simulink model "DC_PlugIn_FastCharging"  (R2023b)
settings: Solver=FixedStepAuto  StartTime=0.0  StopTime=10.0  FixedStep=0.001  RelTol=1e-3
settings Model: Creator=OWNER  LastModifiedBy=OWNER

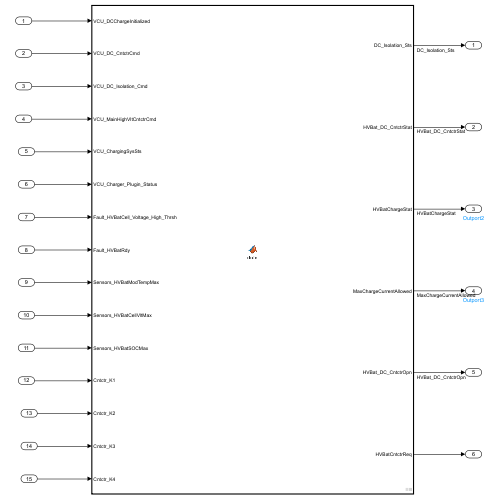
[thumbnail: Simulink's stored preview of the top-level diagram]
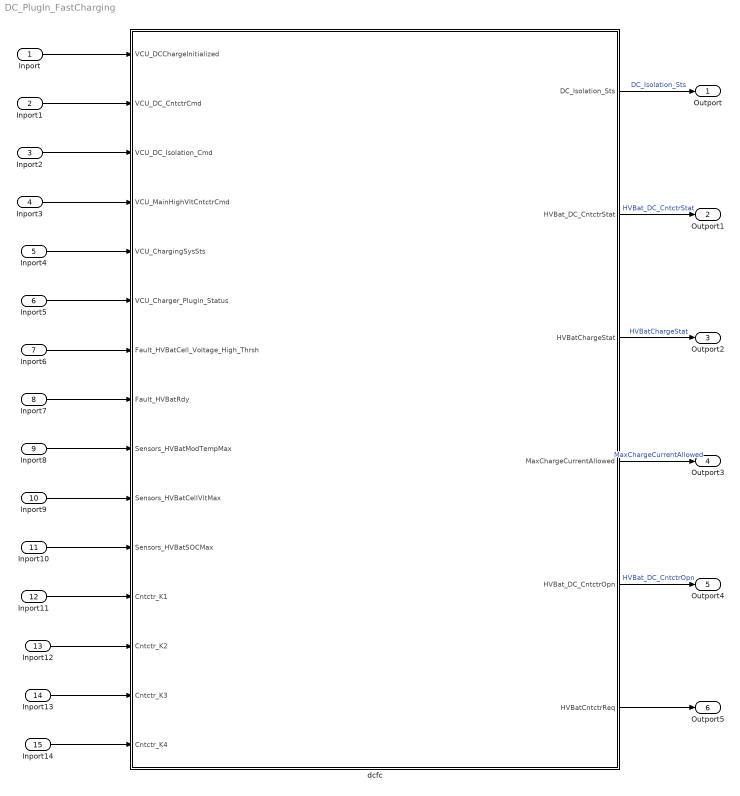
== system DC_PlugIn_FastCharging ==
  Inport : Inport
  Inport1 : Inport  Port=2
  Inport2 : Inport  Port=3
  Inport3 : Inport  Port=4
  Inport4 : Inport  Port=5
  Inport5 : Inport  Port=6
  Inport6 : Inport  Port=7
  Inport7 : Inport  Port=8
  Inport8 : Inport  Port=9
  Inport9 : Inport  Port=10
  Inport10 : Inport  Port=11
  Inport11 : Inport  Port=12
  Inport12 : Inport  Port=13
  Inport13 : Inport  Port=14
  Inport14 : Inport  Port=15
  dcfc : MATLAB Function  TreatAsAtomicUnit=on
  Outport : Outport
  Outport1 : Outport  Port=2
  Outport2 : Outport  Port=3
  Outport3 : Outport  Port=4
  Outport4 : Outport  Port=5
  Outport5 : Outport  Port=6
  wires:
  dcfc/1(DC_Isolation_Sts) -> Outport/1  "DC_Isolation_Sts"
  dcfc/2(HVBat_DC_CntctrStat) -> Outport1/1  "HVBat_DC_CntctrStat"
  dcfc/3(HVBatChargeStat) -> Outport2/1  "HVBatChargeStat"
  dcfc/4(MaxChargeCurrentAllowed) -> Outport3/1  "MaxChargeCurrentAllowed"
  dcfc/5(HVBat_DC_CntctrOpn) -> Outport4/1  "HVBat_DC_CntctrOpn"
  dcfc/6(HVBatCntctrReq) -> Outport5/1
  Inport/1 -> dcfc/1(VCU_DCChargeInitialized)
  Inport1/1 -> dcfc/2(VCU_DC_CntctrCmd)
  Inport2/1 -> dcfc/3(VCU_DC_Isolation_Cmd)
  Inport3/1 -> dcfc/4(VCU_MainHighVltCntctrCmd)
  Inport4/1 -> dcfc/5(VCU_ChargingSysSts)
  Inport7/1 -> dcfc/8(Fault_HVBatRdy)
  Inport6/1 -> dcfc/7(Fault_HVBatCell_Voltage_High_Thrsh)
  Inport5/1 -> dcfc/6(VCU_Charger_Plugin_Status)
  Inport8/1 -> dcfc/9(Sensors_HVBatModTempMax)
  Inport11/1 -> dcfc/12(Cntctr_K1)
  Inport10/1 -> dcfc/11(Sensors_HVBatSOCMax)
  Inport9/1 -> dcfc/10(Sensors_HVBatCellVltMax)
  Inport13/1 -> dcfc/14(Cntctr_K3)
  Inport12/1 -> dcfc/13(Cntctr_K2)
  Inport14/1 -> dcfc/15(Cntctr_K4)

== matlab function DC_PlugIn_FastCharging/dcfc ==
  settings: updateMethod=DISCRETE
  data: DC_Isolation_Sts output; HVBat_DC_CntctrStat output; HVBatChargeStat output; VCU_DCChargeInitialized input; MaxChargeCurrentAllowed output; VCU_DC_CntctrCmd input; VCU_DC_Isolation_Cmd input; VCU_MainHighVltCntctrCmd input; VCU_ChargingSysSts input; VCU_Charger_Plugin_Status input; Fault_HVBatCell_Voltage_High_Thrsh input; Fault_HVBatRdy input; Sensors_HVBatModTempMax input; Sensors_HVBatCellVltMax input; Sensors_HVBatSOCMax input; Cntctr_K1 input; Cntctr_K2 input; Cntctr_K3 input; HVBat_DC_CntctrOpn output; HVBatCntctrReq output; Cntctr_K4 input
function [DC_Isolation_Sts, HVBat_DC_CntctrStat, HVBatChargeStat, MaxChargeCurrentAllowed, HVBat_DC_CntctrOpn, HVBatCntctrReq] ...
    = dcfc(VCU_DCChargeInitialized, VCU_DC_CntctrCmd, VCU_DC_Isolation_Cmd, VCU_MainHighVltCntctrCmd, VCU_ChargingSysSts, VCU_Charger_Plugin_Status, Fault_HVBatCell_Voltage_High_Thrsh, ...
    Fault_HVBatRdy, Sensors_HVBatModTempMax, Sensors_HVBatCellVltMax, Sensors_HVBatSOCMax, Cntctr_K1, Cntctr_K2, Cntctr_K3, Cntctr_K4)
% ===========================
%% INPUTS
% VCU_DC_CntctrCmd - Command from VCU indicating vehicle is plugged into DCFC station and ready to close DCFC contactor (Cntctr_K4) (0 - Open, 1 - Closed, 2 - Impact Open, 3 - Fast Open, 7 - SNA).
% VCU_MainHighVltCntctrCmd - Command from VCU indicating main contactor (Cntctr_K1) is commanded to close (0 - Open, 1 - Closed, 2 - Impact Open, 3 - Fast Open, 7 - SNA).
% Cntctr_K4 - Physical feedback (status of DCFC contactor) (1 - physically closed, 0 - physically open).
% Cntctr_K3 - Physical feedback (status of precharge (+) contactor) (1 - physically closed, 0 - physically open).
% Cntctr_K2 - Physical feedback (status of precharge (-) contactor) (1 - physically closed, 0 - physically open).
% Cntctr_K1 - Physical feedback (status of main contactor) (1 - physically closed, 0 - physically open).
% Fault_HVBatRdy - Indicate if DCFC contactor driver circuit fault or a weld is detected (0 - normal, 1 - at least 1 fault detected).
% VCU_DC_Isolation_Cmd - Command from VCU to disable isolation monitoring when DCFC active (0 - Enable, 1 - Disable).
% VCU_ChargingSysSts - Command from VCU and indicates the status of the charging function (0 - Not Charging, 1 - Charging, 2 - ChargeInterrupted, 3 - ChargeComplete, 7 - SNA).
% VCU_Charger_Plugin_Status - Signal from charge port. True if DCFC connector is plugged in (0 - Charger_Unplugged, 1 - Charger_Plugged_In).
% HVBatPack_Voltage - Current HV pack voltage (V).
% MaxCellVoltage_V - Highest measured cell voltage (V).
% Fault_HVBatCell_Voltage_High_Thrsh - Signal from the BPCM indicating the maximum cell voltage that the battery pack needs to be below in order to become functional. Above this value, the BPCM will set HVBatCntctrReq to 1, and HVBat_DC_CntctrOpn to 1 after appropriate maturation time. If above this value during power up, Fault_HVBatRdy will also be set to 0.
% cellTemperature - All cell temperatures in degC.
% cellVoltage - All cell voltages in V.
% cellSOC - All cell SOCs in percentages.
% ===========================
%% OUTPUTS
% HVBat_DC_CntctrStat - DCFC contactor status (0 - Open, 1 - Closed, 2 - Faulted).
% HVBatChargeStat - Sent out by the BPCM as an indication of its present status (0 - Not Ready, 1 - Ready, 2 - Complete).
% DC_Isolation_Sts - Isolation status for DC charging (0 - Enable, 1 - Disable).
% HVBatMaxCellVltAlld - Max allowable cell voltage (V).
% HVBatMaxPkVltAllwd - Max allowable pack voltage (V).
% MaxChargeCurrentAllowed - Max allowable DCFC current (A).
% HVBatCntctrReq - Request to open contactors (fault/weld) (0 - No request to open, 1 - Request to open).
% HVBat_DC_CntctrOpn - Command to DCFC contactor coil (Not Commanded Open, 1 - Commanded Open).
%% CALIBRATIONS (Constants/Tunable Parameters)
% MaxChargeCurrentDefault - Max allowable DCFC charging current (Default = 30 A).
% Ke_T_HighChrgTempThresholdIn - Upper limit for enabling charging (Default = 50 deg C).
% Ke_T_HighChrgTempThresholdOut - Upper hysteresis threshold (Default = 48 deg C).
% Ke_T_LowChrgTempThresholdIn - Lower limit for enabling charging (Default = -25 deg C).
% Ke_T_LowChrgTempThresholdOut - Lower hysteresis threshold (Default = -23 deg C).
% Ke_U_ChargeCompletionVlt - Voltage threshold for charge completion (Default = 4.14 V).
% Ke_t_DCFC_CntctrOpn - Delay before opening contactor after fault (Default = 1.5 sec).
% ParallelCellNum - Number of parallel cell, which dictates pack current (34).
%% --- Lookup Table for AC Max Charge Current [SOC vs Temp]
SOC = [0 5 10 15 20 25 30 35 40 45 50 55 60 65 70 75 80 85 90 95 100]; % 19 + 2 points
Temp = [-25 -20 -10 0 5 10 20 25 35 40 50]; % 11 points
DCChgCurrentProfile = [ ...
  0.05 0.05 0.05 0.05 0.05 0.05 0.05 0.05 0.05 0.05 0.05 0.05 0.05 0.02 0.02 0.01 0.01 0.01 0.01 0.01 0.00; ...
  0.06 0.06 0.06 0.06 0.06 0.06 0.06 0.06 0.06 0.06 0.06 0.06 0.06 0.02 0.02 0.02 0.02 0.01 0.01 0.01 0.00; ...
  0.45 0.45 0.45 0.45 0.45 0.15 0.15 0.15 0.15 0.09 0.09 0.09 0.09 0.03 0.03 0.03 0.03 0.02 0.02 0.02 0.00; ...
  0.70 0.70 0.70 0.70 0.70 0.70 0.70 0.70 0.70 0.50 0.50 0.50 0.50 0.25 0.25 0.25 0.25 0.10 0.10 0.10 0.00; ...
  0.85 0.85 0.85 0.85 0.85 0.85 0.85 0.85 0.85 0.75 0.75 0.75 0.75 0.63 0.63 0.58 0.58 0.35 0.35 0.20 0.00; ...
  1.00 1.00 1.00 1.00 1.00 1.00 1.00 1.00 1.00 1.00 1.00 1.00 1.00 1.00 1.00 0.90 0.90 0.60 0.60 0.30 0.00; ...
  1.33 1.33 1.33 1.33 1.33 1.33 1.33 1.33 1.33 1.33 1.33 1.33 1.33 1.33 1.33 1.30 1.30 0.80 0.80 0.50 0.00; ...
  1.50 1.50 1.50 1.50 1.50 1.50 1.50 1.50 1.50 1.50 1.50 1.50 1.50 1.50 1.50 1.50 1.50 0.90 0.90 0.60 0.00; ...
  2.17 2.17 2.17 2.17 2.17 2.17 2.17 2.17 2.17 2.17 2.17 2.17 2.17 1.83 1.83 1.50 1.50 0.90 0.90 0.60 0.00; ...
  2.50 2.50 2.50 2.50 2.50 2.50 2.50 2.50 2.50 2.50 2.50 2.50 2.50 2.00 2.00 1.50 1.50 0.90 0.90 0.60 0.00; ...
  1.50 1.50 1.50 1.50 1.50 1.50 1.50 1.50 1.50 1.50 1.50 1.50 1.50 1.50 1.50 1.00 1.00 0.60 0.60 0.48 0.00  ...
];
%% --- Calibration (tunable) ---
% --- Contactor timing calibrations ---
persistent MaxChargeCurrentDefault ...
           Ke_T_HighChrgTempThresholdIn Ke_T_LowChrgTempThresholdIn ...
           Ke_U_ChargeCompletionVlt ...
           ParallelCellNum Ke_t_ChargeCompletionHold  ...
           chargeCompleteFlag overTempFlag ...
           Ke_t_DCFC_CntctrOpn Ke_t_CntctrReqDelay
if isempty(MaxChargeCurrentDefault)
    Ke_t_DCFC_CntctrOpn = 1500;           % 1500 ms - time between HVBat_DC_CntctrOpn and actual coil open
    Ke_t_CntctrReqDelay = 30000;          % 30000 ms - time HVBatCntctrReq must persist before notifying HVBat_DC_CntctrOpn
    Ke_t_ChargeCompletionHold = 300;     % 300 ms
    
    MaxChargeCurrentDefault = 30;        % A (plugin default)
    Ke_T_HighChrgTempThresholdIn = 50;   % degC
    Ke_T_LowChrgTempThresholdIn  = -25;  % degC
    Ke_U_ChargeCompletionVlt = 4.14;     % V per cell held for completion (example)
    ParallelCellNum = 34;
    
    chargeCompleteFlag = false;
    overTempFlag = false;
end
%% --- Persistent runtime state ---
persistent HVBatChargeStat_Aux DC_Isolation_Sts_Aux HVBat_DC_CntctrStat_Aux MaxChargeCurrentAllowed_Aux HVBatChargeTimer ...
           HVBatCntctrReq_Aux HVBat_DC_CntctrOpn_Aux CntctrReqStartTime CntctrOpnStartTime
if isempty(HVBatChargeStat_Aux)
    HVBatChargeStat_Aux = 0;
    DC_Isolation_Sts_Aux = 0;
    HVBat_DC_CntctrStat_Aux = 0;
    MaxChargeCurrentAllowed_Aux = 0;
    HVBatChargeTimer = -1;
    % Contactor request/opn runtime state
    HVBatCntctrReq_Aux = 0;     % immediate request flag
    HVBat_DC_CntctrOpn_Aux = 0;     % "will open within Ke_t_DCFC_CntctrOpn" notification
    
    CntctrReqStartTime = -1;    % when request first asserted
    CntctrOpnStartTime = -1;    % when opn notification first asserted
end
%% Default outputs
    
HVBat_DC_CntctrStat = HVBat_DC_CntctrStat_Aux;
HVBatChargeStat = HVBatChargeStat_Aux;
DC_Isolation_Sts = DC_Isolation_Sts_Aux;
MaxChargeCurrentAllowed = MaxChargeCurrentAllowed_Aux;
HVBat_DC_CntctrOpn = HVBat_DC_CntctrOpn_Aux;
% --- REMOVED Global Fault Detection Block ---
%% ---------- Step: Continuous isolation detection handling ----------
% Requirement: run continuous isolation detection whenever VCU_DC_Isolation_Cmd == 0
% and provide isolation status when DC_Isolation_Disable_Sts = ENABLE.
% Here we model DC_Isolation_Sts = VCU_DC_Isolation_Cmd (1=Disabled, 0=Enabled)    
if VCU_DC_Isolation_Cmd == 1 && VCU_Charger_Plugin_Status == 1 && ~chargeCompleteFlag
    DC_Isolation_Sts_Aux = 1; % DISABLED
else
    DC_Isolation_Sts_Aux = 0; % ENABLED
end
DC_Isolation_Sts = DC_Isolation_Sts_Aux;
%% ---------- Step: Plug detection and readiness ----------
% This block now only handles non-fault states
if VCU_Charger_Plugin_Status == 1 && VCU_DCChargeInitialized == 1 && ~chargeCompleteFlag && ~overTempFlag && Fault_HVBatRdy == 1
    % initial state: not ready until main contactor confirmed closed
    HVBatChargeStat_Aux = 0; % Not Ready
    % main contactor closure commanded by VCU (VCU_MainHighVltCntctrCmd) and confirmed via Cntctr_K1
    % precharge contactors Cntctr_K2,Cntctr_K3 should be open (0) at final close
    if VCU_MainHighVltCntctrCmd == 1 && Cntctr_K1 == 1 && Cntctr_K2 == 0 && Cntctr_K3 == 0 && ~chargeCompleteFlag && ~overTempFlag && Fault_HVBatRdy == 1
        HVBatChargeStat_Aux = 1; % Ready
        MaxChargeCurrentAllowed_Aux = 0;
    end
elseif VCU_Charger_Plugin_Status == 1 && VCU_DCChargeInitialized == 1 && chargeCompleteFlag && ~overTempFlag
        MaxChargeCurrentAllowed_Aux = 0;
        HVBat_DC_CntctrStat_Aux = 0;   % Open
        HVBatChargeStat_Aux = 6;       % Complete
else
    % unplugged: reset readiness and clear DC-specific states
    HVBatChargeStat_Aux = 0;
    HVBat_DC_CntctrStat_Aux = 0;
    MaxChargeCurrentAllowed_Aux = 0;
end
%% ---------- Step: DC contactor commanded by VCU and BPCM reporting ----------
% VCU commands DC contactor close via VCU_DC_CntctrCmd.
% When VCU commanded close and actual feedback Cntctr_K4 == 1, BPCM reports Closed.
% If commanded closed but Cntctr_K4 never closes and a fault is detected, BPCM reports Faulted.
if VCU_DC_CntctrCmd == 1
    % --- VCU requests contactor closure ---
    if chargeCompleteFlag || overTempFlag
        % Charging is inhibited: force open
        HVBat_DC_CntctrStat_Aux = 0;  % Open
        if overTempFlag
            HVBatChargeStat_Aux = 3;  % Charge disallowed
        end
    else
        % Charging allowed: reflect physical feedback
        if Cntctr_K4 == 1
            HVBat_DC_CntctrStat_Aux = 1;  % Closed
        else
            HVBat_DC_CntctrStat_Aux = 0;  % Open
        end
    end
else
    % --- VCU does NOT request closure ---
    % Report physical state only (no command implied)
    if Cntctr_K4 == 1
        HVBat_DC_CntctrStat_Aux = 1;  % Closed (anomalous but truthful)
    else
        HVBat_DC_CntctrStat_Aux = 0;  % Open
    end
end
%% ---------- Step: Charging handshake and DCFC charging stage ----------
% Preconditions for handshake
handshake_ok = (HVBatChargeStat_Aux == 1) && ...      % Ready
               (DC_Isolation_Sts_Aux == 1) && ...    % Isolation disabled
               (HVBat_DC_CntctrStat_Aux == 1) && ... % DC contactor closed
               (VCU_ChargingSysSts == 1);             % Charger active
% Handshake transition (one-way)
if handshake_ok
    HVBatChargeStat_Aux = 2; % Charge allow
end
%% ---------- Signal aliases ----------
Vmax        = Sensors_HVBatCellVltMax;
Temp_actual = Sensors_HVBatModTempMax;
SOC_actual  = Sensors_HVBatSOCMax;
Vreset      = Ke_U_ChargeCompletionVlt;
%% ---------- Over-temperature hysteresis ----------
if overTempFlag
    if (Temp_actual <= (Ke_T_HighChrgTempThresholdIn - 5)) && ...
       (Temp_actual >= (Ke_T_LowChrgTempThresholdIn  + 5))
        overTempFlag = false;
    end
end
%% ---------- Normal DC Charging ----------
if (HVBatChargeStat_Aux == 2) && ...
   (VCU_ChargingSysSts == 1) && ...
   (Vmax < Vreset) && ...
   (~chargeCompleteFlag) && ...
   (~overTempFlag)
    % DCFC current profile
    MaxChargeCurrentAllowed_Aux = ...
        ParallelCellNum * interp2( ...
            SOC, Temp, DCChgCurrentProfile, ...
            SOC_actual, Temp_actual);
    % Maintain closed contactor during charging
    HVBat_DC_CntctrStat_Aux = 1;
%% ---------- Charge Completion Detection ----------
elseif (HVBatChargeStat_Aux == 2) && ...
       (VCU_ChargingSysSts == 1 || VCU_ChargingSysSts == 3) && ...
       (Vmax >= Vreset) && ...
       (~chargeCompleteFlag) && ...
       (~overTempFlag)
    if HVBatChargeTimer < 0
        HVBatChargeTimer = 0;
    else
        HVBatChargeTimer = HVBatChargeTimer + 1; % 1 ms tick
    end
    if HVBatChargeTimer >= Ke_t_ChargeCompletionHold
        MaxChargeCurrentAllowed_Aux = 0;
        HVBatChargeStat_Aux = 6;       % Charge complete
        DC_Isolation_Sts_Aux = 0;      % Re-enable isolation
        chargeCompleteFlag = true;
    end
%% ---------- Voltage fell before completion ----------
elseif (HVBatChargeStat_Aux == 2) && (Vmax < Vreset)
    HVBatChargeTimer = -1;
%% ---------- Over-temperature inhibit ----------
elseif (Temp_actual >= Ke_T_HighChrgTempThresholdIn) || ...
       (Temp_actual <= Ke_T_LowChrgTempThresholdIn)
    % Charging inhibit only (safety layer handles contactors)
    MaxChargeCurrentAllowed_Aux = 0;
    overTempFlag = true;
    HVBatChargeStat_Aux = 3; % Charge disallowed
end
%% ---------- Step: Global Fault Override (with request + open timers) ----------
% Fault condition that requires contactor open
fault_active = (Fault_HVBatRdy == 0) || (overTempFlag) || (Sensors_HVBatCellVltMax >= Fault_HVBatCell_Voltage_High_Thrsh);
if fault_active
    %% -------- Stage 1: Immediate Request --------
    HVBatCntctrReq_Aux = 1;
    if CntctrReqStartTime < 0
        CntctrReqStartTime = 0;
    else
        CntctrReqStartTime = CntctrReqStartTime + 1; % 1 ms tick
    end
    %% -------- Stage 2: Open Notification (Latched) --------
    if CntctrReqStartTime >= Ke_t_CntctrReqDelay
        HVBat_DC_CntctrOpn_Aux = 1;   % latch: will open
    end
    if HVBat_DC_CntctrOpn_Aux
        if CntctrOpnStartTime < 0
            CntctrOpnStartTime = 0;
        else
            CntctrOpnStartTime = CntctrOpnStartTime + 1; % 1 ms tick
        end
    end
    %% -------- Stage 3: Forced Open --------
    if HVBat_DC_CntctrOpn_Aux && (CntctrOpnStartTime >= Ke_t_DCFC_CntctrOpn)
        % Commanded-open / faulted state
        HVBat_DC_CntctrStat_Aux = 2;     % Faulted
        HVBatChargeStat_Aux     = 3;     % Charge disallowed
        DC_Isolation_Sts_Aux    = 0;     % Isolation enforced
        MaxChargeCurrentAllowed_Aux = 0; % No charge current
    end
else
    % no fault: clear all timers/flags and reset DC_Cntctr_Opn_Aux
    HVBatCntctrReq_Aux = 0;
    HVBat_DC_CntctrOpn_Aux = 0;
    CntctrReqStartTime = -1;
    CntctrOpnStartTime = -1;
    % If it was previously marked faulted/disallow, allow the state machine to re-evaluate
    if HVBat_DC_CntctrStat_Aux == 2 && Cntctr_K4 == 0 % DC contactor faulted
        HVBat_DC_CntctrStat_Aux = 0;
    end
end
%% ---------- Assign outputs ----------
HVBat_DC_CntctrStat = HVBat_DC_CntctrStat_Aux;
HVBatChargeStat = HVBatChargeStat_Aux;
DC_Isolation_Sts = DC_Isolation_Sts_Aux;
MaxChargeCurrentAllowed = MaxChargeCurrentAllowed_Aux;
HVBat_DC_CntctrOpn = HVBat_DC_CntctrOpn_Aux;   
HVBatCntctrReq = HVBatCntctrReq_Aux;   
% make sure no NaN
if isnan(MaxChargeCurrentAllowed), MaxChargeCurrentAllowed = 0; end
end
